simulink model "bldc_Hall"  (R2022a)
settings: Solver=VariableStepDiscrete  StartTime=0.0  StopTime=2  RelTol=1e-5
InitFcn:
  | f=2000;
  | m=0.8;
  | Ts=1/f;
  | Vdc=48;
libraries: spsDCVoltageSourceLib x1, simulink x1, spsPermanentMagnetSynchronousMachineLib x1, spsUniversalBridgeLib x1, spspowerguiLib x1
settings Model: Creator=XieXW  LastModifiedBy=XieXW

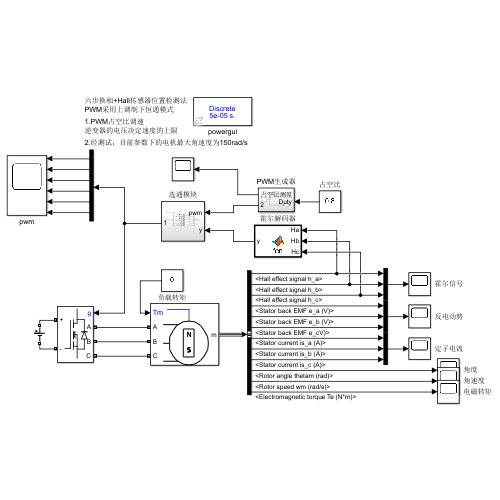
[thumbnail: Simulink's stored preview of the top-level diagram]
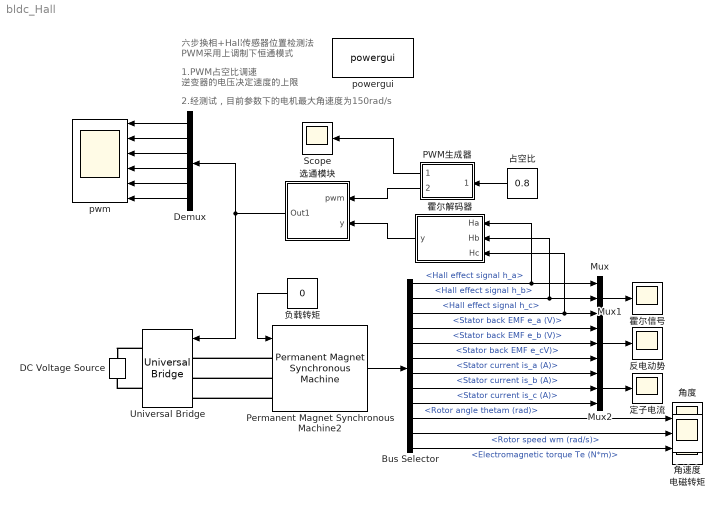
== system bldc_Hall ==
  note: 2.经测试，目前参数下的电机最大角速度为150rad/s
  note: 1.PWM占空比调速
      | 逆变器的电压决定速度的上限
  note: 六步换相+Hall传感器位置检测法
      | PWM采用上调制下恒通模式
  Bus Selector : BusSelector  OutputSignals=Hall effect signal h_a,Hall effect signal h_b,Hall effect signal h_c,Stator back EMF e_a (V),Stator back EMF e_b (V),Stator back EMF e_cV),Stator current is_a (A),Stator current is_b (A),Stator current is_c (A),Rotor angle thetam (rad),Rotor speed wm (rad/s),Electromagnetic torque Te (N*m)
  DC Voltage Source : spsDCVoltageSourceLib/DC Voltage Source  Amplitude=Vdc  Measurements=None
  Demux : Demux  Outputs=6
  Mux : Mux  Inputs=3
  Mux1 : Mux  Inputs=3
  Mux2 : Mux  Inputs=3
  PWM生成器 : Subsystem
  Permanent Magnet Synchronous Machine2 : spsPermanentMagnetSynchronousMachineLib/Permanent Magnet Synchronous Machine  NbPhases=3  FluxDistribution=Trapezoidal  RotorType=Round  MechanicalLoad=Torque Tm  PresetModel=No  ShowDetailedParameters=on  MeasurementBus=off  Resistance=0.0485  Inductance=8.5e-3  dqInductances=[8.5e-3,8.5e-3]  La=0.000395  MachineConstant=Flux linkage established by magnets (V.s)  Flux=0.1194  VoltageCst=25.0071  TorqueCst=0.2388  Flat=120  Mechanical=[0.0027 0.0124924 1 0]  PolePairs=4  InitialConditions=[0,0, 0,0]  InitialConditions5ph=[0 0 0 0 0 0]  RefAngle=Aligned with phase A axis (original Park)  IterativeDiscreteModel=Trapezoidal non iterative  TsBlock=-1  TsPowergui=0
  Scope : Scope
  Universal Bridge : spsUniversalBridgeLib/Universal Bridge  Arms=3  SnubberResistance=1e5  SnubberCapacitance=inf  Device=MOSFET / Diodes  Ron=1e-3  Lon=0  ForwardVoltages="[  0  0  ]"  ForwardVoltage=0  GTOparameters=[ 10e-6 , 20e-6 ]  IGBTparameters=[ 1e-6 , 2e-6 ]  Measurements=None  Measurements_2=None  converterType=Rectifier
  powergui : spspowerguiLib/powergui  Priority=1  SimulationMode=Discrete  SampleTime=50e-6  frequency=60  Iterations=50  frequencyindice=0  Pbase=100e6  ErrMax=1e-4  UnitsV=kV  UnitsW=MW  buscounter=0  FunctionMessages=off  echomessages=off  EnableUseOfTLC=off  CurrentSourceSwitches=off  DisableSnubberDevices=off  DisableRonSwitches=off  DisableVfSwitches=off  DisplayEquations=off  AutomaticDiscreteSolvers=off  SolverType=Tustin/Backward Euler (TBE)  Interpol=off  ExternalGateDelay=off  methode=off  Ts=100  x0status=blocks  SPID=on  SwTol=0  HookPort=off  NonlinearTolerance=1e-4  nMaxIteration=100  ContinueOnMaxIteration=off  RestoreLinks=warning  ResistiveCurrentMeasurement=off  Frange=[0:2:500]  Ylog=off  Xlog=on  ShowGrid=off  save=off  variable=ZData  structure=0  ZoomFFT=off  StartTime=0.0  cycles=1  DisplayStyle=1  fundamental=60  FreqAxis=off  MaxFrequency=1000  frequencyindicesteady=1  RmsSteady=1  display=off
  pwm : Scope  NumInputPorts=6
  占空比 : Constant  Value=0.8
  反电动势 : Scope
  定子电流 : Scope
  电磁转矩 : Scope
  角度 : Scope
  角速度 : Scope
  负载转矩 : Constant  Value=0
  选通模块 : Subsystem
  霍尔信号 : Scope
  霍尔解码器 : MATLAB Function  TreatAsAtomicUnit=on
  wires:
  Mux/1 -> 霍尔信号/1
  Bus Selector/5 -> Mux1/2  "<Stator back EMF e_b (V)>"
  Bus Selector/6 -> Mux1/3  "<Stator back EMF e_cV)>"
  Mux1/1 -> 反电动势/1
  Bus Selector/11 -> 角速度/1  "<Rotor speed wm (rad/s)>"
  负载转矩/1 -> Permanent Magnet Synchronous Machine2/1
  Permanent Magnet Synchronous Machine2/1 -> Bus Selector/1
  Bus Selector/4 -> Mux1/1  "<Stator back EMF e_a (V)>"
  Bus Selector/1 -> Mux/1, 霍尔解码器/1(Ha)  "<Hall effect signal h_a>"
  Bus Selector/2 -> Mux/2, 霍尔解码器/2(Hb)  "<Hall effect signal h_b>"
  Bus Selector/3 -> Mux/3, 霍尔解码器/3(Hc)  "<Hall effect signal h_c>"
  Bus Selector/7 -> Mux2/1  "<Stator current is_a (A)>"
  Bus Selector/8 -> Mux2/2  "<Stator current is_b (A)>"
  Bus Selector/9 -> Mux2/3  "<Stator current is_c (A)>"
  Mux2/1 -> 定子电流/1
  Bus Selector/12 -> 电磁转矩/1  "<Electromagnetic torque Te (N*m)>"
  霍尔解码器/1(y) -> 选通模块/2(y)
  PWM生成器/2(Out1) -> 选通模块/1(pwm)
  选通模块/1(Out1) -> Demux/1, Universal Bridge/1
  Demux/1 -> pwm/1
  Demux/2 -> pwm/2
  Demux/3 -> pwm/3
  Demux/4 -> pwm/4
  Demux/5 -> pwm/5
  Demux/6 -> pwm/6
  Bus Selector/10 -> 角度/1  "<Rotor angle thetam (rad)>"
  PWM生成器/1(占空比测量) -> Scope/1
  占空比/1 -> PWM生成器/1(Duty)
  connections:
  Universal Bridge/RConn1 -- DC Voltage Source/RConn1
  Universal Bridge/RConn2 -- DC Voltage Source/LConn1
  Permanent Magnet Synchronous Machine2/LConn1 -- Universal Bridge/LConn1
  Permanent Magnet Synchronous Machine2/LConn2 -- Universal Bridge/LConn2
  Permanent Magnet Synchronous Machine2/LConn3 -- Universal Bridge/LConn3

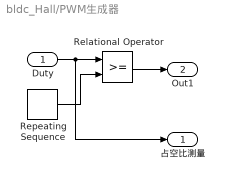
== system bldc_Hall/PWM生成器 ==
  Duty : Inport
  Relational Operator : RelationalOperator  OutDataTypeStr=boolean  RndMeth=Simplest  InputSameDT=off
  Repeating Sequence : simulink/Sources/Repeating Sequence  rep_seq_t=[0 0.001]  rep_seq_y=[0 1]
  占空比测量 : Outport
  Out1 : Outport  Port=2
  wires:
  Relational Operator/1 -> Out1/1
  Duty/1 -> 占空比测量/1, Relational Operator/1
  Repeating Sequence/1 -> Relational Operator/2

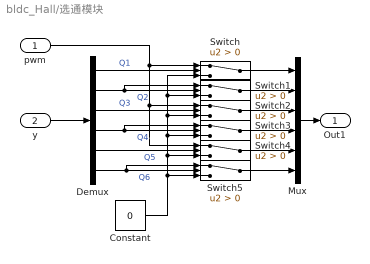
== system bldc_Hall/选通模块 ==
  pwm : Inport
  y : Inport  Port=2
  Constant : Constant  Value=0
  Demux : Demux  Outputs=6
  Mux : Mux  Inputs=6
  Switch{,1..5} (6 alike) : Switch  Criteria=u2 > Threshold  SaturateOnIntegerOverflow=off  InputSameDT=off
  Out1 : Outport
  wires:
  y/1 -> Demux/1
  Demux/1 -> Switch/2  "Q1"
  Demux/3 -> Switch2/2  "Q3"
  Demux/4 -> Switch3/1, Switch3/2  "Q4"
  Demux/5 -> Switch4/2  "Q5"
  Demux/6 -> Switch5/1, Switch5/2  "Q6"
  pwm/1 -> Switch/1, Switch4/1, Switch2/1
  Constant/1 -> Switch5/3, Switch4/3, Switch3/3, Switch2/3, Switch1/3, Switch/3
  Demux/2 -> Switch1/1, Switch1/2  "Q2"
  Switch2/1 -> Mux/3
  Switch3/1 -> Mux/4
  Switch4/1 -> Mux/5
  Switch5/1 -> Mux/6
  Switch1/1 -> Mux/2
  Switch/1 -> Mux/1
  Mux/1 -> Out1/1

== matlab function bldc_Hall/霍尔解码器 ==
  data: Ha input; Hb input; y output; Hc input
function y = fcn(Ha, Hb, Hc)

if isequal([Ha,Hb,Hc], [0,0,1])
    Q1=0; Q2=0; Q3=0; Q4=1; Q5=1; Q6=0; % CB
elseif isequal([Ha,Hb,Hc], [0,1,0])
    Q1=0; Q2=1; Q3=1; Q4=0; Q5=0; Q6=0; % BA
elseif isequal([Ha,Hb,Hc], [0,1,1])
    Q1=0; Q2=1; Q3=0; Q4=0; Q5=1; Q6=0; % CA
elseif isequal([Ha,Hb,Hc], [1,0,0])
    Q1=1; Q2=0; Q3=0; Q4=0; Q5=0; Q6=1; % AC
elseif isequal([Ha,Hb,Hc], [1,0,1])
    Q1=1; Q2=0; Q3=0; Q4=1; Q5=0; Q6=0; % AB
elseif isequal([Ha,Hb,Hc], [1,1,0])
    Q1=0; Q2=0; Q3=1; Q4=0; Q5=0; Q6=1; % BC
else
    Q1=0; Q2=0; Q3=0; Q4=0; Q5=0; Q6=0; 
end

y = [Q1, Q2, Q3, Q4, Q5, Q6];
